simulink model "training_data_switching"  (R2025b)
settings: Solver=ode1be  StartTime=0.0  StopTime=5/60  FixedStep=1/3840  RelTol=1e-3
values from neighbouring files (symbols this model uses):
  trigger_samples = 80    [LG_faults_rework.m]    (also in Small_DataSet.m; Training_Dataset_toolbox_livescript_pipeline_1.m; Training_Dataset_toolbox_livescript_pipeline_2.m; Training_Dataset_toolbox_livescript_pipeline_3.m)
settings Model: Creator=faizshaikh  LastModifiedBy=faizshaikh

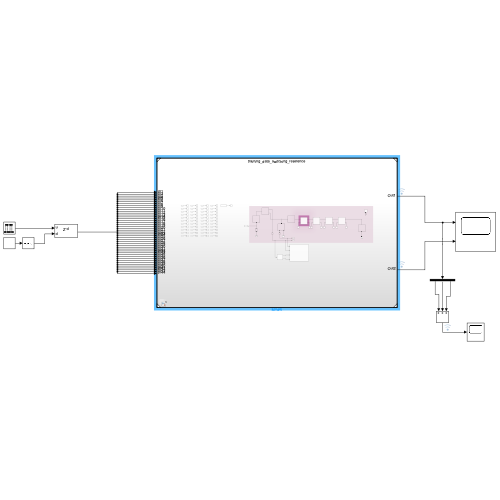
[thumbnail: Simulink's stored preview of the top-level diagram]
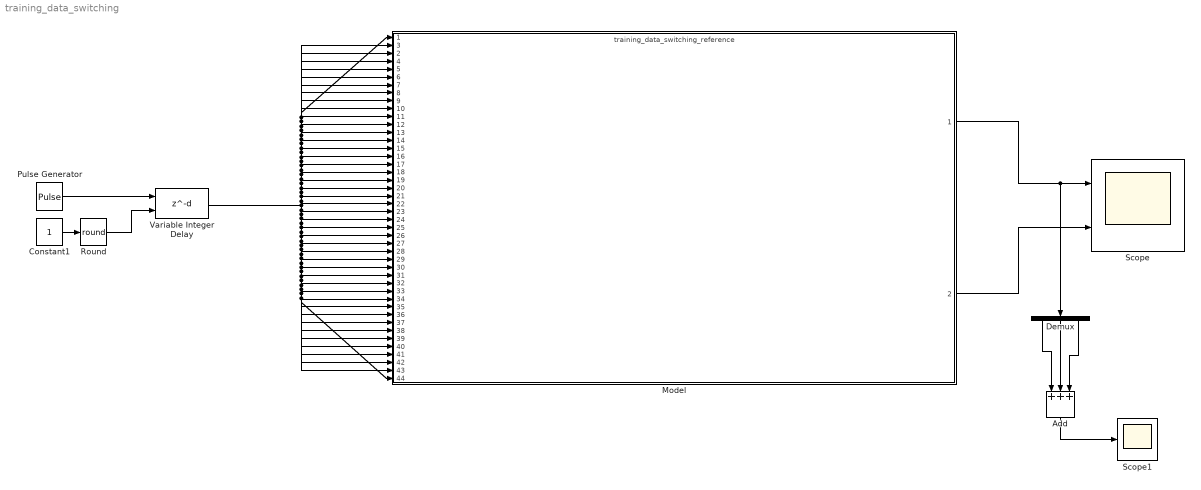
== system training_data_switching ==
  Add : Sum  Inputs=+++
  Constant1 : Constant  SampleTime=1/3840
  Demux : Demux  Outputs=3
  Model : ModelReference  ModelNameDialog=training_data_switching_reference.slx  SimulationMode=Normal  ModelReferenceVersion=1.21
      settings: PortSchema="{\"entries\":[{\"content\":{\"sides\":[{\"content\":{\"connectorIds\":[\"In1\",\"In3\",\"In2\",\"In4\",\"In5\",\"In6\",\"In7\",\"In8\",\"In9\",\"In10\",\"In11\",\"In12\",\"In13\",\"In14\",\"In15\",\"In16\",\"In17\",\"In18\",\"In19\",\"In20\",\"In21\",\"In22\",\"In23\",\"In24\",\"In25\",\"In26\",\"In27\",\"In28\",\"In29\",\"In30\",\"In31\",\"In32\",\"In33\",\"In34\",\"In35\",\"In36\",\"In37\",\"In38\",\"In39\",\"In40\",\"In41\",\"In42\",\"In43\",\"In44\"]},\"type\":\"ConnectorPlacement.EquallySpacedRectSide\",\"uuid\":\"53a54c55-af73-4118-857d-086d9ec6a0ff\"},{\"content\":{\"connectorIds\":[\"Out1\",\"Out2\"],\"side\":\"RIGHT\"},\"type\":\"ConnectorPlacement.EquallySpacedRectSide\",\"uuid\":\"680475f5-ca90-46be-bcd5-2f466c996b83\"},{\"content\":{\"side\":\"TOP\"},\"type\":\"ConnectorPlacement.EquallySpacedRectSide\",\"uuid\":\"194ee6f4-ae29-4b22-91d2-fa1414a36eee\"}]},\"type\":\"ConnectorPlacement.EquallySpacedConnector\",\"uuid\":\"1ef3efce-1c6b-4919-af77-a01c8e883a89\"}],\"packageUris\":[\"http://schema.mathworks.com/mf0/Connector/R2020b\"],\"version\":\"1.0\"}"
  Pulse Generator : DiscretePulseGenerator  Period=10  PulseWidth=5  PhaseDelay=trigger_samples  SampleTime=1/3840
  Round : Rounding  Operator=round
  Scope : Scope  NumInputPorts=2
      settings: ActiveDisplayYMinimum=-135.8164428383993  ActiveDisplayYMaximum=135.68395879392511
  Scope1 : Scope
      settings: ActiveDisplayYMinimum=-8.79296635503124E-14  ActiveDisplayYMaximum=8.08242361927114E-14
  Variable Integer Delay : Delay  DelayLengthSource=Input port  SampleTime=1/3840
      settings: InputPortMap=u0,p1
  wires:
  Model/1 -> Scope/1, Demux/1
  Model/2 -> Scope/2
  Pulse Generator/1 -> Variable Integer Delay/1
  Variable Integer Delay/1 -> Model/44, Model/43, Model/42, Model/41, Model/40, Model/39, Model/38, Model/37, Model/36, Model/35, Model/34, Model/33, Model/32, Model/31, Model/30, Model/29, Model/28, Model/27, Model/26, Model/25, Model/24, Model/23, Model/21, Model/20, Model/19, Model/18, Model/17, Model/16, Model/15, Model/14, Model/13, Model/12, Model/11, Model/10, Model/9, Model/7, Model/6, Model/2, Model/3, Model/1, Model/4, Model/5, Model/8, Model/22
  Constant1/1 -> Round/1
  Round/1 -> Variable Integer Delay/2
  Demux/2 -> Add/2
  Demux/1 -> Add/1
  Demux/3 -> Add/3
  Add/1 -> Scope1/1
